simulink model "FlapDuuuuuragControlSimulatorForFriends"  (R2024b)
settings: Solver=VariableStepAuto  StartTime=0.0  StopTime=20  RelTol=1e-3
undefined symbols (not defined in the file): Asymptote, Body_Diameter, Body_Length, csv, DiscIntNeverNeededParam, Dragx, Dragy, Dry_Mass, Empty_Motor_Mass, Fin_Area, Flap_Length, Flap_width, flaps, Integral, Integral_Motor_Curve, Motorx, Motory, num_Flaps, optimize, Pressure, Propellent_Mass, Proportional, Rail_Angle, Temp, time_at_final, time_constants_to_final, wind_direction, wind_speed, wind_Z, Y_int_offset
libraries: simulink x4, simulink_extras x3, slpidlib x2, aerolibwind2 x2, aerolibutil x1, sharedtransform x1, eeGeneralControl x1
(part 2 of 2)

== system FlapDuuuuuragControlSimulatorForFriends/User Parameters/Control System/Controller (coppied from L2)/Double Integrator ==
  In2 : Inport
  Discrete-Time Integrator1 : DiscreteIntegrator  SampleTime=-1  ICPrevOutput=DiscIntNeverNeededParam  ICPrevScaledInput=DiscIntNeverNeededParam
  Discrete-Time Integrator2 : DiscreteIntegrator  SampleTime=-1  ICPrevOutput=DiscIntNeverNeededParam  ICPrevScaledInput=DiscIntNeverNeededParam
  Discrete-Time Integrator3 : DiscreteIntegrator  SampleTime=-1  ICPrevOutput=DiscIntNeverNeededParam  ICPrevScaledInput=DiscIntNeverNeededParam
  Filtered Derivative (Discrete or Continuous) : eeGeneralControl/Filtered Derivative (Discrete or Continuous)  K=1  T=10  B=inf  A=-inf  minRatio=10  init_option=Inherited from block input  x0=0  Ts=-1
      settings: LibrarySourceBlock=|
      | ee_sl_lib/General Control/Filtered Derivative
      | (Discrete or Continuous)
  Gain1 : Gain  Gain=-0.003
  Gain2 : Gain  Gain=-0.005
  Gain3 : Gain  Gain=-0.002
  Gain4 : Gain  Gain=-0.005
  Saturation1 : Saturate  UpperLimit=0.9879  LowerLimit=0
  Sum2 : Sum  Inputs=++++
  Out2 : Outport
  wires:
  In2/1 -> Gain2/1, Gain1/1, Gain4/1, Gain3/1
  Sum2/1 -> Saturation1/1
  Gain1/1 -> Discrete-Time Integrator1/1
  Gain3/1 -> Discrete-Time Integrator3/1
  Saturation1/1 -> Out2/1
  Gain4/1 -> Filtered Derivative (Discrete or Continuous)/1
  Discrete-Time Integrator2/1 -> Sum2/3
  Filtered Derivative (Discrete or Continuous)/1 -> Sum2/4
  Gain2/1 -> Sum2/1
  Discrete-Time Integrator3/1 -> Discrete-Time Integrator2/1
  Discrete-Time Integrator1/1 -> Sum2/2

== system FlapDuuuuuragControlSimulatorForFriends/User Parameters/Control System/Controller (coppied from L2)/Gain Scheduling ==
  In1 : Inport
  Constant4 : Constant
  Step : Step  Time=5  Before=-0.01  After=-0.05  SampleTime=0
  Step1 : Step  Time=5  Before=-0.005  After=-0.1  SampleTime=0
  Step2 : Step  Time=5  Before=-0.005  After=-0.005  SampleTime=0
  Tuned Controller : slpidlib/PID Controller  Controller=PID  Form=Parallel  TimeDomain=Discrete-time  UseExternalTs=off  SampleTime=0.01  IntegratorMethod=Forward Euler  FilterMethod=Forward Euler  ControllerParametersSource=external  P=-0.005  I=-0.005  UseKiTs=off  D=-0.005  UseExternalDerivativeSource=off  N=1  UseFilter=on  TunerSelectOption=Transfer Function Based (PID Tuner App)  InitialConditionSource=internal  InitialConditionForIntegrator=0  InitialConditionForFilter=0  DifferentiatorICPrevScaledInput=0  ExternalReset=none  TrackingMode=off  Kt=1  LimitOutput=on  SatLimitsSource=internal  UpperSaturationLimit=pi/2  LowerSaturationLimit=0  LinearizeAsGain=off  AntiWindupMode=back-calculation  Kb=1  LimitIntegrator=off  UpperIntegratorSaturationLimit=pi/2  LowerIntegratorSaturationLimit=0  POutMin=[]  POutMax=[]  IOutMin=[]  IOutMax=[]  DOutMin=[]  DOutMax=[]  NOutMin=[]  NOutMax=[]  SumOutMin=[]  SumOutMax=[]  SaturationOutMin=[]  SaturationOutMax=[]  PParamMin=[]  PParamMax=[]  IParamMin=[]  IParamMax=[]  DParamMin=[]  DParamMax=[]  NParamMin=[]  NParamMax=[]  KbParamMin=[]  KbParamMax=[]  KtParamMin=[]  KtParamMax=[]  KbOutMin=[]  KbOutMax=[]  KtOutMin=[]  KtOutMax=[]  IntegratorOutMin=[]  IntegratorOutMax=[]  FilterOutMin=[]  FilterOutMax=[]  SumI1OutMin=[]  SumI1OutMax=[]  SumI2OutMin=[]  SumI2OutMax=[]  SumI3OutMin=[]  SumI3OutMax=[]  SumI4OutMin=[]  SumI4OutMax=[]  SumDOutMin=[]  SumDOutMax=[]  DifferentiatorOutMin=[]  DifferentiatorOutMax=[]  FilterDiffOutCoefMin=[]  FilterDiffOutCoefMax=[]  ReciprocalOutMin=[]  ReciprocalOutMax=[]  SumDenOutMin=[]  SumDenOutMax=[]  SumNumOutMin=[]  SumNumOutMax=[]  DivideOutMin=[]  DivideOutMax=[]  UdiffTsProdOutMin=[]  UdiffTsProdOutMax=[]  NTsProdOutMin=[]  NTsProdOutMax=[]  UintegralTsProdOutMin=[]  UintegralTsProdOutMax=[]  UngainTsProdOutMin=[]  UngainTsProdOutMax=[]  ClampingZeroOutDataTypeStr=Inherit: Inherit via back propagation  ClampingZeroOutMin=[]  ClampingZeroOutMax=[]  FilterDenConstantOutDataTypeStr=Inherit: Inherit via back propagation  FilterDenConstantOutMin=[]  FilterDenConstantOutMax=[]  PCopyOutDataTypeStr=Inherit: Inherit via back propagation  PCopyOutMin=[]  PCopyOutMax=[]  NCopyOutDataTypeStr=Inherit: Inherit via back propagation  NCopyOutMin=[]  NCopyOutMax=[]  IntegratorContinuousStateAttributes=''  IntegratorStateMustResolveToSignalObject=off  IntegratorRTWStateStorageClass=Auto  FilterContinuousStateAttributes=''  FilterStateMustResolveToSignalObject=off  FilterRTWStateStorageClass=Auto  ParallelPVariant=ExternalParameters  IdealPVariant=Disabled  IVariant=ExternalParameters  DVariant=ExternalParameters  IntegratorVariant=Discrete  SatVariant=Enabled  AWVariant=BackCalculation  PCopyVariant=Disabled  TRVariant=Disabled  FdbkBlocksVariant=Forward  IdealPFdbkVariant=Disabled  SatFdbkVariant=Disabled  DerivativeFilterVariant=ForwardEulerFilter  NVariant=ExternalParameters  NCopyVariant=Disabled  FilterICVariant=InternalICsFilter  IntegratorICVariant=InternalICs  ExternalResetVariant=Disabled  TRSumVariant=Passthrough  SumFdbkVariant=Disabled  SumVariant=Sum_PID  TsampFilterVariant=InternalTs  TsampNgainVariant=Passthrough  TsampIntegralVariant=Disabled_SignalSpec  ExternalSaturationOutDataTypeStr=Inherit: Same as second input  DerivativeSourceVariant=ErrorSignal  PreIntVariant=InternalPreInt
  Out1 : Outport
  wires:
  In1/1 -> Tuned Controller/1
  Tuned Controller/1 -> Out1/1
  Constant4/1 -> Tuned Controller/5
  Step2/1 -> Tuned Controller/4
  Step1/1 -> Tuned Controller/3
  Step/1 -> Tuned Controller/2

== system FlapDuuuuuragControlSimulatorForFriends/User Parameters/Control System/Controller (coppied from L2)/PID ==
  note: update this to max rotation of motor(90deg)
  note: The L3 has interference at about
      |  73 degrees, roughly 2/5 pi
  In1 : Inport
  Input : Inport  Port=2
  Constant : Constant  Commented=on  Value=pi/2
  Constant1 : Constant  Value=0
  Constant2 : Constant  Value=pi/2
  PID Controller : slpidlib/PID Controller  Controller=PI  Form=Parallel  TimeDomain=Discrete-time  UseExternalTs=off  SampleTime=0.01  IntegratorMethod=Forward Euler  FilterMethod=Forward Euler  ControllerParametersSource=internal  P=Proportional  I=Integral  UseKiTs=off  D=-0.0005  UseExternalDerivativeSource=off  N=1  UseFilter=on  TunerSelectOption=Transfer Function Based (PID Tuner App)  InitialConditionSource=internal  InitialConditionForIntegrator=0  InitialConditionForFilter=0  DifferentiatorICPrevScaledInput=0  ExternalReset=none  TrackingMode=off  Kt=1  LimitOutput=on  SatLimitsSource=external  UpperSaturationLimit=pi/2  LowerSaturationLimit=0  LinearizeAsGain=on  AntiWindupMode=none  Kb=1  LimitIntegrator=off  UpperIntegratorSaturationLimit=inf  LowerIntegratorSaturationLimit=-inf  POutMin=[]  POutMax=[]  IOutMin=[]  IOutMax=[]  DOutMin=[]  DOutMax=[]  NOutMin=[]  NOutMax=[]  SumOutMin=[]  SumOutMax=[]  SaturationOutMin=[]  SaturationOutMax=[]  PParamMin=[]  PParamMax=[]  IParamMin=[]  IParamMax=[]  DParamMin=[]  DParamMax=[]  NParamMin=[]  NParamMax=[]  KbParamMin=[]  KbParamMax=[]  KtParamMin=[]  KtParamMax=[]  KbOutMin=[]  KbOutMax=[]  KtOutMin=[]  KtOutMax=[]  IntegratorOutMin=[]  IntegratorOutMax=[]  FilterOutMin=[]  FilterOutMax=[]  SumI1OutMin=[]  SumI1OutMax=[]  SumI2OutMin=[]  SumI2OutMax=[]  SumI3OutMin=[]  SumI3OutMax=[]  SumI4OutMin=[]  SumI4OutMax=[]  SumDOutMin=[]  SumDOutMax=[]  DifferentiatorOutMin=[]  DifferentiatorOutMax=[]  FilterDiffOutCoefMin=[]  FilterDiffOutCoefMax=[]  ReciprocalOutMin=[]  ReciprocalOutMax=[]  SumDenOutMin=[]  SumDenOutMax=[]  SumNumOutMin=[]  SumNumOutMax=[]  DivideOutMin=[]  DivideOutMax=[]  UdiffTsProdOutMin=[]  UdiffTsProdOutMax=[]  NTsProdOutMin=[]  NTsProdOutMax=[]  UintegralTsProdOutMin=[]  UintegralTsProdOutMax=[]  UngainTsProdOutMin=[]  UngainTsProdOutMax=[]  ClampingZeroOutDataTypeStr=Inherit: Inherit via back propagation  ClampingZeroOutMin=[]  ClampingZeroOutMax=[]  FilterDenConstantOutDataTypeStr=Inherit: Inherit via back propagation  FilterDenConstantOutMin=[]  FilterDenConstantOutMax=[]  PCopyOutDataTypeStr=Inherit: Inherit via back propagation  PCopyOutMin=[]  PCopyOutMax=[]  NCopyOutDataTypeStr=Inherit: Inherit via back propagation  NCopyOutMin=[]  NCopyOutMax=[]  IntegratorContinuousStateAttributes=''  IntegratorStateMustResolveToSignalObject=off  IntegratorRTWStateStorageClass=Auto  FilterContinuousStateAttributes=''  FilterStateMustResolveToSignalObject=off  FilterRTWStateStorageClass=Auto  ParallelPVariant=InternalParameters  IdealPVariant=Disabled  IVariant=InternalParameters  DVariant=Disabled  IntegratorVariant=Discrete  SatVariant=External  AWVariant=Passthrough  PCopyVariant=Disabled  TRVariant=Disabled  FdbkBlocksVariant=Forward  IdealPFdbkVariant=Disabled  SatFdbkVariant=Disabled  DerivativeFilterVariant=Disabled  NVariant=Disabled  NCopyVariant=Disabled_SignalSpec  FilterICVariant=Disabled  IntegratorICVariant=InternalICs  ExternalResetVariant=Disabled  TRSumVariant=Passthrough  SumFdbkVariant=Disabled  SumVariant=Sum_PI  TsampFilterVariant=InternalTs  TsampNgainVariant=Passthrough  TsampIntegralVariant=Disabled_SignalSpec  ExternalSaturationOutDataTypeStr=Inherit: Same as second input  DerivativeSourceVariant=Disabled  PreIntVariant=InternalPreInt
  Rate Transition : RateTransition
  Subtract : Sum  Inputs=+-
  Subtract1 : Sum  Inputs=+-
  Out1 : Outport
  wires:
  Constant/1 -> ?
  Constant1/1 -> Subtract1/1
  Input/1 -> Subtract/2, Subtract1/2
  In1/1 -> PID Controller/1
  Subtract/1 -> PID Controller/2
  Subtract1/1 -> PID Controller/3
  PID Controller/1 -> Rate Transition/1
  Rate Transition/1 -> Out1/1
  Constant2/1 -> Subtract/1

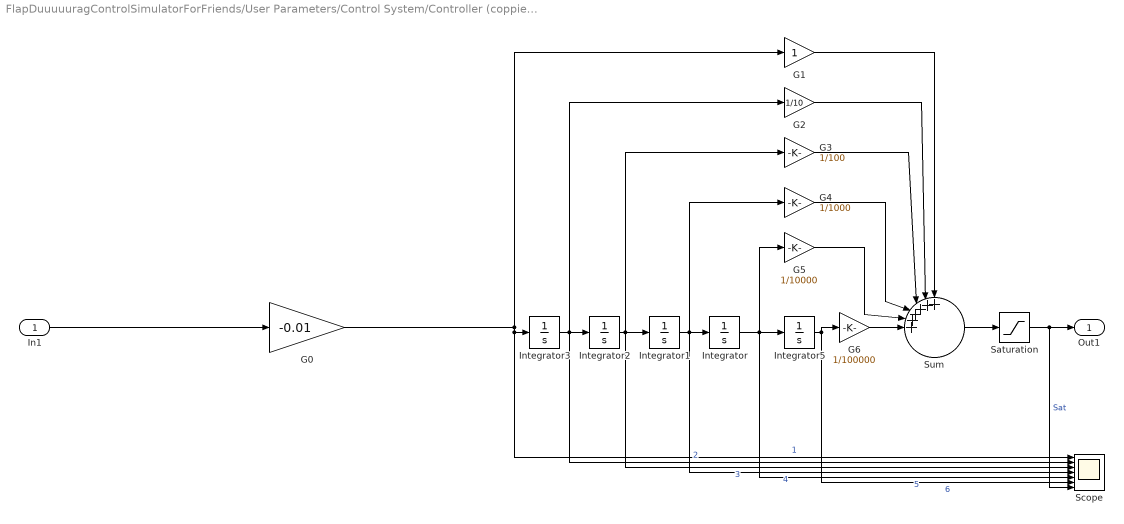
== system FlapDuuuuuragControlSimulatorForFriends/User Parameters/Control System/Controller (coppied from L2)/Shennanigans ==
  In1 : Inport
  G0 : Gain  Gain=-0.01
  G1 : Gain
  G2 : Gain  Gain=1/10
  G3 : Gain  Gain=1/100
  G4 : Gain  Gain=1/1000
  G5 : Gain  Gain=1/10000
  G6 : Gain  Gain=1/100000
  Integrator{,1..3,5} (5 alike) : Integrator
  Saturation : Saturate  UpperLimit=pi/2  LowerLimit=0
  Scope : Scope  NumInputPorts=7
  Sum : Sum  Inputs=++++++|||||
  Out1 : Outport
  wires:
  G0/1 -> Integrator3/1, Scope/1, G1/1  "1"
  In1/1 -> G0/1
  Integrator3/1 -> G2/1, Integrator2/1, Scope/2  "2"
  Integrator2/1 -> G3/1, Integrator1/1, Scope/3  "3"
  Integrator1/1 -> G4/1, Integrator/1, Scope/4  "4"
  Integrator/1 -> G5/1, Integrator5/1, Scope/5  "5"
  Saturation/1 -> Scope/7, Out1/1  "Sat"
  Sum/1 -> Saturation/1
  Integrator5/1 -> G6/1, Scope/6  "6"
  G6/1 -> Sum/6
  G1/1 -> Sum/1
  G2/1 -> Sum/2
  G3/1 -> Sum/3
  G4/1 -> Sum/4
  G5/1 -> Sum/5

== system FlapDuuuuuragControlSimulatorForFriends/User Parameters/Control System/Controller (coppied from L2)/Shennanigans Part 2 ==
  In1 : Inport
  Out1 : Outport

== matlab function FlapDuuuuuragControlSimulatorForFriends/Dynamics/Drag Calculations/2022-2023 CFD/MATLAB Function ==
  data: body_diam_in input; Fd_lbf output size=3; flap_length_in input; flap_width_in input; number_flaps input; flap_angle_deg input; temp_K input; velocity_ft_s input; pressure_Pa input
function Fd_lbf = flapsmodel(body_diam_in,flap_length_in,flap_width_in,number_flaps,flap_angle_deg,temp_K,velocity_ft_s,pressure_Pa)
%args: diameter, flap len, width, inches
%number_flaps: integer
%temperature in kelvin
%pressure in pascals
%velocity in ft./s
%flap_angle in degrees

%returns: drag force according to 2023's CFD results in lbf

rho=(2.758e-3).*pressure_Pa./temp_K;
rho=rho.*0.062428./32.174; %convert to lbm./ft3
Aprofile=pi.*(body_diam_in./2).^2;
A_airbrakes_max=number_flaps.*flap_length_in.*flap_width_in;
mu_imp=(1.458e-6).*temp_K.^(3./2)./(temp_K+110.4);
mu_imp=mu_imp.*0.224809./10.7639;


if flap_angle_deg <7.325
    MR_L = Aprofile.*(rho).^2.*(velocity_ft_s).^2./(mu_imp).^2;
    Fd_lbf= (MR_L.*10.^-11+1.7689); %sketchy at this level
elseif flap_angle_deg < 30
    MR_L = (Aprofile+A_airbrakes_max.*sin(7.325.*pi./180)).*(rho).^2.*(velocity_ft_s).^2./(mu_imp).^2;
    MR_H = (Aprofile+A_airbrakes_max.*sin(30.*pi./180)).*(rho).^2.*(velocity_ft_s).^2./(mu_imp).^2;
    Fd_lbf = ((30-flap_angle_deg).*(MR_L.*10.^-11+1.7689))./30+((flap_angle_deg-30).*(MR_H.*10.^-11+2.0931))./30;
elseif flap_angle_deg < 60
    MR_L = (Aprofile+A_airbrakes_max.*sin(30.*pi./180)).*(rho).^2.*(velocity_ft_s).^2./(mu_imp).^2;
    MR_H = (Aprofile+A_airbrakes_max.*sin(60.*pi./180)).*(rho).^2.*(velocity_ft_s).^2./(mu_imp).^2;
    Fd_lbf = ((60-flap_angle_deg).*(MR_L.*10.^-11+2.0931))./30+((flap_angle_deg-30).*(MR_H.*10.^-11+2.6925))./30;
elseif flap_angle_deg <= 90
    MR_L = (Aprofile+A_airbrakes_max.*sin(60.*pi./180)).*(rho).^2.*(velocity_ft_s).^2./(mu_imp).^2;
    MR_H = (Aprofile+A_airbrakes_max.*sin(90.*pi./180)).*(rho).^2.*(velocity_ft_s).^2./(mu_imp).^2;
    Fd_lbf = ((90-flap_angle_deg).*(MR_L.*10.^-11+2.6925))./30+((flap_angle_deg-30).*(MR_H.*10.^-11+2.0551))./30;
else
    error('Flaps Out of Bounds')
end

== stateflow chart FlapDuuuuuragControlSimulatorForFriends/Chart ==
  state Pre_Launch
    entry:
    doJostling = 1;
    doGravity = 0;
    exit:
    doJostling = 0;
  state Burn
    entry:
    doMotor = 1;
    doGravity = 1;
    exit:
    doMotor = 0;
  state Post_Burnout
    entry:
    doControl = 1;
    exit:
    doControl = 0;
  state Recovery
    entry:
    inRecovery = 1;
  (default) -> Burn
  Post_Burnout -> Recovery : [Vz<=0]
  Burn -> Post_Burnout : [motorForce<=0 & Vz>10]
  Pre_Launch -> Burn : [launchButton==1]
  data: launchButton input; Vz input; doMotor output; doControl output; motorForce input; doJostling output; doGravity output; inRecovery output
